simulink model "psbarrester"  (Simulink 6.0)
settings: Solver=ode23tb  SolverMode=SingleTasking  StartTime=0.0  StopTime=.1  FixedStep=40e-6  RelTol=1e-4
libraries: powerlib2 x17, simulink x1
settings Model: Creator=patrice  LastModifiedBy=batserve  ExtModeTrigMode=oneshot  ExtModeArmWhenConnect=off  ExtModeAutoUpdateStatusClock=off
settings DataIOCC: LimitDataPoints=off  SignalLoggingName=sigsOut  OutputTimes=0.00001
settings OptimizationCC: BooleanDataType=off
settings DebuggingCC: AlgebraicLoopMsg=none  SolverPrmCheckMsg=none
settings HardwareCC: TargetUnknown=on
settings RTWCC: TemplateMakefile=grt_unix.tmf

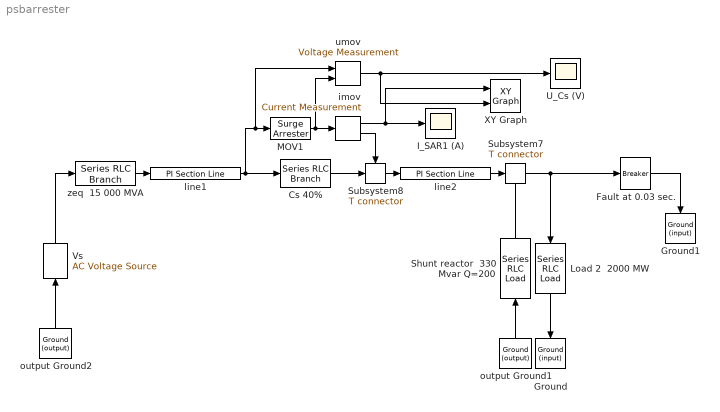
== system psbarrester ==
  " MOV1" : powerlib2/Elements/Surge Arrester  Tag=PoWeRsYsTeMbLoCk  x1=185e3  x2=30  x3=500  x4=[.955 50]  x5=[1.0 25]  x6=[.9915 16.5]  mesure=None  PSBOutputType=1
  Cs 40% : powerlib2/Elements/Series RLC Branch  Tag=PoWeRsYsTeMbLoCk  a=0  b=0  c=101.4e-6  mesure=None  PSBOutputType=1
  Fault at 0.03 sec. : powerlib2/Elements/Breaker  Tag=PoWeRsYsTeMbLoCk  a=1  c=0  rs=inf  cs=0  times="[ 30e-3  300e-3 ]"  Ts=0  comext=off  mesure=None  PSBOutputType=1
  Ground : powerlib2/Connectors/Ground (input)  Tag=PoWeRsYsTeMbLoCk  Orientation=down
  Ground1 : powerlib2/Connectors/Ground (input)  Tag=PoWeRsYsTeMbLoCk  Orientation=down
  I_SAR1 (A) : Scope
      settings: TickLabels=on  TimeRange=0.1  YMin=-5000  YMax=10000  DataFormat=Array  MaxDataPoints=500000
  Load 2  2000 MW : powerlib2/Elements/Series RLC Load  Tag=PoWeRsYsTeMbLoCk  Orientation=down  a=735e3/sqrt(3)  b=60  c=2000e6/3  d=0  e=0  mesure=None  PSBOutputType=1
  Shunt reactor  330 Mvar Q=200 : powerlib2/Elements/Series RLC Load  Tag=PoWeRsYsTeMbLoCk  Orientation=up  a=735e3/sqrt(3)  b=60  c=330e6/3/200  d=330e6/3  e=0  mesure=None  PSBOutputType=1
  Subsystem7 : powerlib2/Connectors/T connector  Tag=PoWeRsYsTeMbLoCk  PSBOutputType=1
  Subsystem8 : powerlib2/Connectors/T connector  Tag=PoWeRsYsTeMbLoCk  PSBOutputType=1
  U_Cs (V) : Scope
      settings: TickLabels=on  TimeRange=0.1  YMin=-200000  YMax=200000  DataFormat=Array  MaxDataPoints=500000
  Vs : powerlib2/Electrical Sources/AC Voltage Source  Tag=PoWeRsYsTeMbLoCk  Orientation=up  A=735e3/sqrt(3)*sqrt(2)  P=0  F=60  stime=0  mesure=None  PSBOutputType=1
  XY Graph : simulink/Sinks/XY Graph  xmin=-6000  xmax=6000  ymin=-2e5  ymax=2e5  st=-1
  imov : powerlib2/Measurements/Current Measurement  Tag=PoWeRsYsTeMmEaSuReMeNt  PhasorSimulation=off  OutputType=Magnitude  PSBOutputType=01  PSBequivalent=0
  line1 : powerlib2/Elements/PI Section Line  Tag=PoWeRsYsTeMbLoCk  f=60  a=0.011  b=0.8674e-3  c=13.41e-9  d=100  e=2  mesure=None  PSBOutputType=1
  line2 : powerlib2/Elements/PI Section Line  Tag=PoWeRsYsTeMbLoCk  f=60  a=0.011  b=0.8674e-3  c=13.41e-9  d=100  e=2  mesure=None  PSBOutputType=1
  output Ground1 : powerlib2/Connectors/Ground (output)  Tag=PoWeRsYsTeMbLoCk  Orientation=up  PSBOutputType=1
  output Ground2 : powerlib2/Connectors/Ground (output)  Tag=PoWeRsYsTeMbLoCk  Orientation=up  PSBOutputType=1
  umov : powerlib2/Measurements/Voltage Measurement  Tag=PoWeRsYsTeMmEaSuReMeNt  PhasorSimulation=off  OutputType=Magnitude  PSBOutputType=0  PSBequivalent=0
  zeq  15 000 MVA : powerlib2/Elements/Series RLC Branch  Tag=PoWeRsYsTeMbLoCk  a=3.6  b=95.5e-3  c=inf  mesure=None  PSBOutputType=1
  wires:
  " MOV1"/1 -> umov/2, imov/1
  Subsystem8/1 -> line2/1
  Vs/1 -> zeq  15 000 MVA/1
  output Ground2/1 -> Vs/1
  zeq  15 000 MVA/1 -> line1/1
  imov/2 -> Subsystem8/Enable
  Cs 40%/1 -> Subsystem8/1
  line1/1 -> umov/1, " MOV1"/1, Cs 40%/1
  Shunt reactor  330 Mvar Q=200/1 -> Subsystem7/Enable
  output Ground1/1 -> Shunt reactor  330 Mvar Q=200/1
  line2/1 -> Subsystem7/1
  Load 2  2000 MW/1 -> Ground/1
  Subsystem7/1 -> Fault at 0.03 sec./1, Load 2  2000 MW/1
  umov/1 -> U_Cs (V)/1, XY Graph/2
  imov/1 -> I_SAR1 (A)/1, XY Graph/1
  Fault at 0.03 sec./1 -> Ground1/1
